simulink model "Feedback_State"  (R2018b)
settings: Solver=VariableStepAuto  StartTime=0.0  StopTime=7  RelTol=1e-3
settings Model: Creator=Mostafa Hamidifard  LastModifiedBy=User

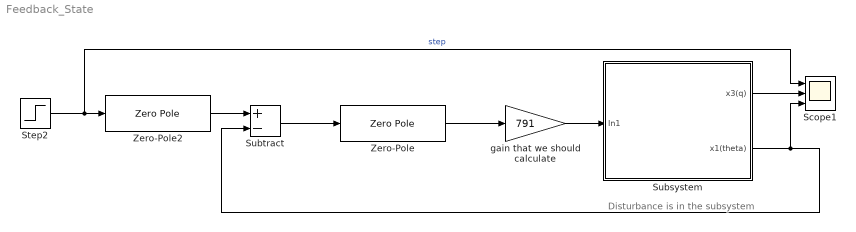
== system Feedback_State ==
  note: Disturbance is in the subsystem
  Scope1 : Scope  NumInputPorts=3
  Step2 : Step  SampleTime=0
  Subsystem : Subsystem
  Subtract : Sum  Inputs=+-
  Zero-Pole : ZeroPole  Zeros=[-2 -2]  Poles=[-25.47 0]
  Zero-Pole2 : ZeroPole  Zeros=[]  Poles=-4  Gain=4
  gain that we should calculate : Gain  Gain=791
  wires:
  gain that we should calculate/1 -> Subsystem/1(In1)
  Subsystem/2(x1(theta)) -> Subtract/2, Scope1/3
  Subtract/1 -> Zero-Pole/1
  Zero-Pole/1 -> gain that we should calculate/1
  Step2/1 -> Zero-Pole2/1, Scope1/1  "step"
  Subsystem/1(x3(q)) -> Scope1/2
  Zero-Pole2/1 -> Subtract/1

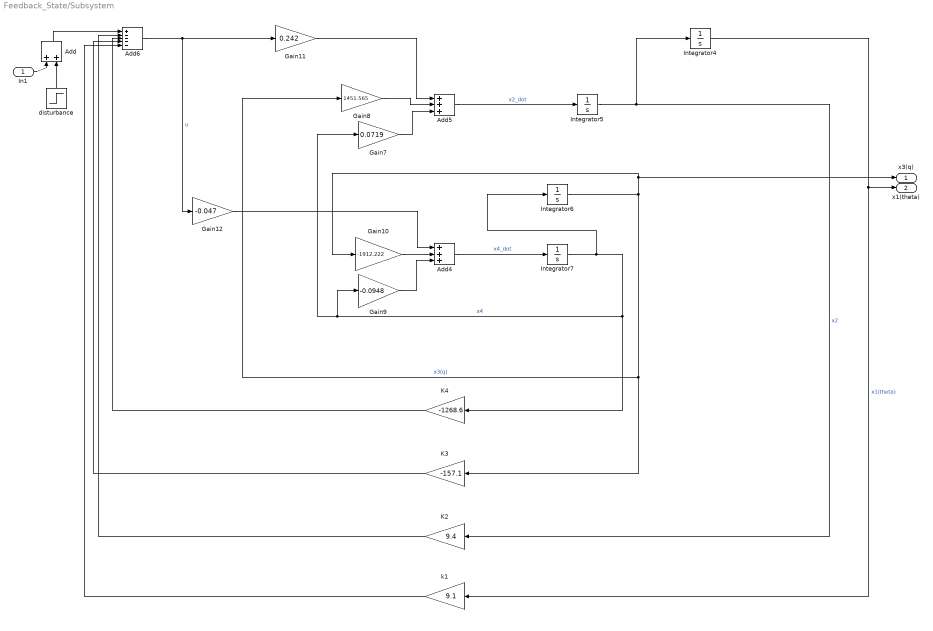
== system Feedback_State/Subsystem ==
  In1 : Inport
  Add : Sum
  Add4 : Sum  Inputs=+++
  Add5 : Sum  Inputs=+++
  Add6 : Sum  Inputs=+----
  Gain10 : Gain  Gain=-1912.222
  Gain11 : Gain  Gain=0.242
  Gain12 : Gain  Gain=-0.047
  Gain7 : Gain  Gain=0.0719
  Gain8 : Gain  Gain=1451.565
  Gain9 : Gain  Gain=-0.0948
  Integrator{4..7} (4 alike) : Integrator
  K2 : Gain  Gain=9.4
  K3 : Gain  Gain=-157.1
  K4 : Gain  Gain=-1268.6
  disturbance : Step  SampleTime=0
  k1 : Gain  Gain=9.1
  x3(q) : Outport
  x1(theta) : Outport  Port=2
  wires:
  Gain12/1 -> Add4/1
  Integrator7/1 -> Integrator6/1, Gain7/1, Gain9/1, K4/1  "x4"
  Gain7/1 -> Add5/3
  Integrator6/1 -> Gain8/1, K3/1, Gain10/1, x3(q)/1  "x3(q)"
  Gain10/1 -> Add4/2
  Gain9/1 -> Add4/3
  K3/1 -> Add6/4
  Add6/1 -> Gain11/1, Gain12/1  "u"
  Gain11/1 -> Add5/1
  Gain8/1 -> Add5/2
  Add4/1 -> Integrator7/1  "x4_dot"
  Integrator5/1 -> K2/1, Integrator4/1  "x2"
  Integrator4/1 -> k1/1, x1(theta)/1  "x1(theta)"
  K4/1 -> Add6/3
  Add5/1 -> Integrator5/1  "x2_dot"
  k1/1 -> Add6/5
  K2/1 -> Add6/2
  In1/1 -> Add/1
  Add/1 -> Add6/1
  disturbance/1 -> Add/2
